simulink model "Closed_Loop"  (R2018b)
settings: Solver=VariableStepAuto  StartTime=0.0  StopTime=10  RelTol=1e-3
values from neighbouring files (symbols this model uses):
  K = place(A,B,p)    [Master.m]
settings Model: Creator=Cam  LastModifiedBy=Cam

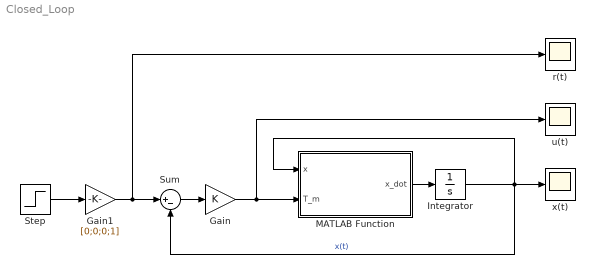
== system Closed_Loop ==
  Gain : Gain  Gain=K
  Gain1 : Gain  Gain=[0;0;0;1]
  Integrator : Integrator  InitialCondition=[0;0;0;.1]
  MATLAB Function : MATLAB Function  TreatAsAtomicUnit=on
  Step : Step  SampleTime=0
  Sum : Sum  Inputs=|+-
  "r(t) " : Scope
  u(t) : Scope
  "x(t) " : Scope
  wires:
  MATLAB Function/1(x_dot) -> Integrator/1
  Integrator/1 -> Sum/2, MATLAB Function/1(x), "x(t) "/1  "x(t)"
  Step/1 -> Gain1/1
  Sum/1 -> Gain/1
  Gain/1 -> u(t)/1, MATLAB Function/2(T_m)
  Gain1/1 -> "r(t) "/1, Sum/1

== matlab function Closed_Loop/MATLAB Function ==
  data: x input; x_dot output; T_m input
function x_dot  = botEOM(x, T_m)

%% Variables
g = 32.174;   %gravity
weight_1=1.1/16;    %weight of wheel, lbf
weight_2=1.63-2*weight_1;       %weight of body, lbf
m_1 = weight_1/g; %mass of wheel, slug
m_2 = weight_2/g; %mass of body
r_1 = 2.55/2; %radius of wheel
r_2 = 1.028; %distance from center of wheel to c.g. of body
I_1 = m_1*r_1^2; %moment of inertia of wheel slug*in^2
I_2 = 1; %moment of inertia of body

m_eff =  m_1 + m_2 + (I_1/r_1^2); %effective mass
I_eff = m_2*r_2^2 + I_2; %effective moment of inertia
b_1 = 0; %damping coefficient from rolling resistance due to translation of x
b_2 = 0; %damping coefficient relative from rolling between wheels to body (theta 2-theta1)

%% matrices
A1 = [m_eff -m_2*r_2*cos(x(4)) 0 0
     -m_2*r_2*cos(x(4)) I_eff 0 0
      0 0 1 0
      0 0 0 1];
A2 = [-T_m/r_1 - (b_2/r_1^2)*x(1) - (b_2/r_1)*x(2) - b_1*x(1) - m_2*r_2*x(2)^2*sin(x(4))
    T_m - (b_2/r_1)*x(1) - b_2*x(2) + m_2*r_2*g*sin(x(4))
    x(1)
    x(2)];

x_dot = inv(A1)*A2;
